simulink model "lab2simulink"  (R2018b)
settings: Solver=FixedStepAuto  StartTime=0.0  StopTime=3.0  FixedStep=0.01  RelTol=1e-3
values from neighbouring files (symbols this model uses):
  h = 0.01    [lab2.m]
  z2 = z1 / 2    [lab2.m]    (also in lab2.mat = -8.3)
undefined symbols (not defined in the file or in its folder): averageTau
settings Model: Creator=mert  LastModifiedBy=mert

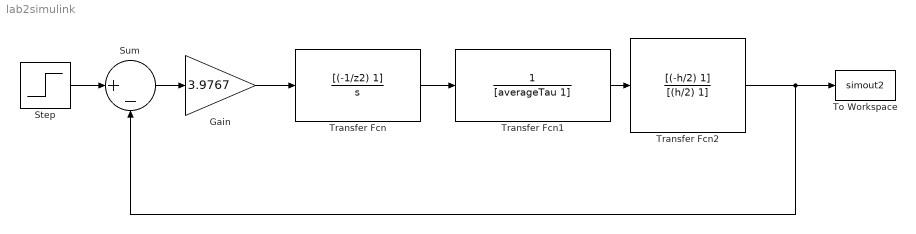
== system lab2simulink ==
  Gain : Gain  Gain=3.9767
  Step : Step  Time=0  After=10  SampleTime=0
  Sum : Sum  Inputs=|+-
  To Workspace : ToWorkspace  VariableName=simout2  SaveFormat=Timeseries  SampleTime=-1
  Transfer Fcn : TransferFcn  Numerator=[(-1/z2) 1]  Denominator=[1 0]
  Transfer Fcn1 : TransferFcn  Denominator=[averageTau 1]
  Transfer Fcn2 : TransferFcn  Numerator=[(-h/2) 1]  Denominator=[(h/2) 1]
  wires:
  Gain/1 -> Transfer Fcn/1
  Sum/1 -> Gain/1
  Transfer Fcn1/1 -> Transfer Fcn2/1
  Step/1 -> Sum/1
  Transfer Fcn/1 -> Transfer Fcn1/1
  Transfer Fcn2/1 -> To Workspace/1, Sum/2
